simulink model "sistema"  (R2023a)
settings: Solver=ode23t  StartTime=0.0  StopTime=140  MaxStep=1E-3  RelTol=1e-3
settings Model: LastModifiedBy=Kami Valle
settings DataIOCC: ReturnWorkspaceOutputs=off  TimeSaveName=t
settings DebuggingCC: AlgebraicLoopMsg=none  ArtificialAlgebraicLoopMsg=none  MaxConsecutiveZCsMsg=none
settings RTWCC: GPUComputeCapability=5.0

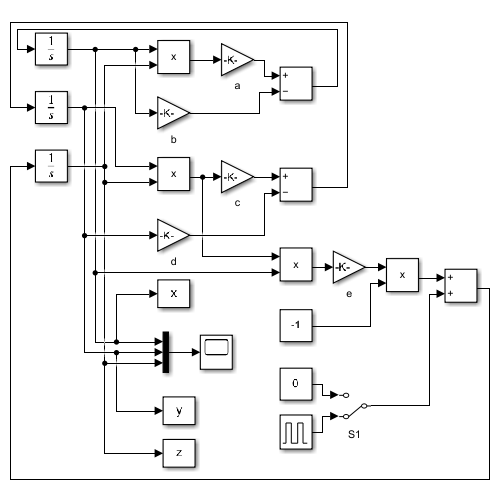
[thumbnail: Simulink's stored preview of the top-level diagram]
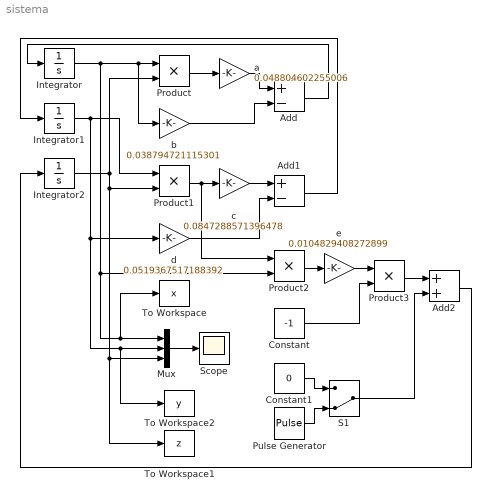
== system sistema ==
  Add : Sum  Inputs=+-
  Add1 : Sum  Inputs=+-
  Add2 : Sum
  Constant : Constant  Value=-1
  Constant1 : Constant  Value=0
  Integrator : Integrator  InitialCondition=0.751260178
  Integrator1 : Integrator  InitialCondition=0.261998584
  Integrator2 : Integrator  InitialCondition=1
  Mux : Mux  Inputs=3
  Product{,1..3} (4 alike) : Product
  Pulse Generator : DiscretePulseGenerator  PulseType=Time based  Amplitude=0.01  Period=150  PulseWidth=10  PhaseDelay=85
  S1 : ManualSwitch  CurrentSetting=0
  Scope : Scope
  To Workspace : ToWorkspace  VariableName=x  SampleTime=-1
  To Workspace1 : ToWorkspace  VariableName=z  SampleTime=-1
  To Workspace2 : ToWorkspace  VariableName=y  SampleTime=-1
  a : Gain  Gain=0.048804602255006
  b : Gain  Gain=0.038794721115301
  c : Gain  Gain=0.0847288571396478
  d : Gain  Gain=0.0519367517188392
  e : Gain  Gain=0.0104829408272899
  wires:
  Integrator/1 -> Mux/1, To Workspace/1, Product2/2, b/1, Product/1
  Integrator2/1 -> To Workspace1/1, Mux/3, Product1/2, Product/2
  Product/1 -> a/1
  a/1 -> Add/1
  b/1 -> Add/2
  Integrator1/1 -> To Workspace2/1, Mux/2, d/1, Product1/1
  Product1/1 -> Product2/1, c/1
  c/1 -> Add1/1
  d/1 -> Add1/2
  Product2/1 -> e/1
  e/1 -> Product3/1
  Constant/1 -> Product3/2
  Product3/1 -> Add2/1
  Add/1 -> Integrator/1
  Add1/1 -> Integrator1/1
  Add2/1 -> Integrator2/1
  Mux/1 -> Scope/1
  Constant1/1 -> S1/1
  Pulse Generator/1 -> S1/2
  S1/1 -> Add2/2
